simulink model "Controller"  (R2015a)
settings: Solver=ode3  SolverMode=SingleTasking  StartTime=0.0  StopTime=100  FixedStep=T_sim  RelTol=1e-3
PreLoadFcn:
  | LoadLibraries
values from neighbouring files (symbols this model uses):
  a = 10.26    [SetupComplete.m]
  A_x = 0.015    [SetupComplete.m]
  A_y = A_x    (= 0.015)    [SetupComplete.m]
  A_z = 0.16    [SetupComplete.m]
  C_d0 = 0.001193    [SetupComplete.m]
  C_x = 1.2    [SetupComplete.m]
  C_y = C_x    (= 1.2)    [SetupComplete.m]
  C_z = 2.2    [SetupComplete.m]
  CG_0 = [0,0,0.02]'    [SetupComplete.m]
  eta_23 = deg2rad(-1.42)    [Run3Copter.m]
  g = 9.81    [SetupComplete.m]
  h = 0.08    [SetupComplete.m]
  h_M = 0.064    [SetupComplete.m]
  I_BAC_0 = [ Ix,0,Ixz;0,Iy,0;Ixz,0,Iz]    [SetupComplete.m]
  Initial_Omegas = [1;1;1]*Omega_hover    [Run3Copter.m]
  l = 0.3450    (= 0.345)    [NDI_components.m]    (also in SetupComplete.m; robust_controller.m)
  l_arm = 0.264    [SetupComplete.m]
  m = 3.51    [SetupComplete.m]
  m_0 = 2.61    [SetupComplete.m]
  m_M = 0.300    (= 0.3)    [SetupComplete.m]
  R = 0.1778    [SetupComplete.m]    (also in robust_controller.m = eye(4))
  rho = 1.15    [SetupComplete.m]
  sigma = b*c/(pi*R)    (= 0.107416159567)    [SetupComplete.m]
  theta_0 = 0.38397    [SetupComplete.m]
  theta_1 = -0.2967    [SetupComplete.m]
  v_i0 = sqrt( 1/3*m*g/(2*rho*pi*R^2)  )    [SetupComplete.m]
undefined symbols (not defined in the file or in its folder): DOWN_0, EAST_0, Motor, NORTH_0, P_0, Prop, Q_0, R_0, Throttle_Hover, U_0, V_0, v_i_adim, Vx_adim, Vz_adim, W_0
undefined symbols (not defined in the file): Initial_Torques, J_FA, J_T, Rotation_sign, Tau_motors
libraries: XXCopter x39, simulink x35, vrlib x15, simulink_extras x7, aerolib6dofsys x2, qcatlib x2, dspinverses x2
(part 3 of 10)

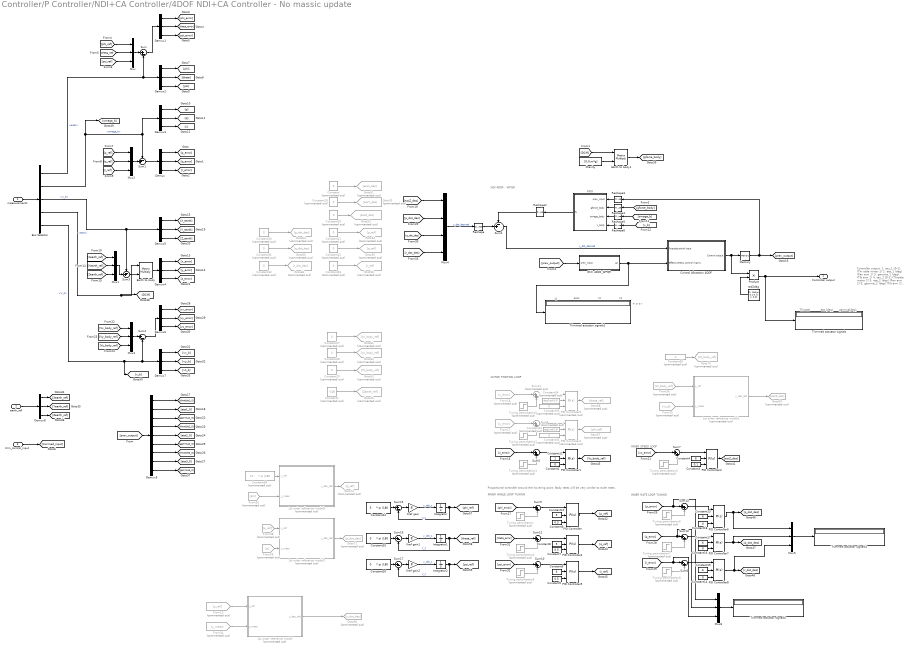
== system Controller/P Controller/NDI+CA Controller/4DOF NDI+CA Controller - No massic update ==
  note: NDI 4DOF - WPQR
  note: INNER SPEED LOOP
  note: INNER ANGLE LOOP TUNING
  note: INNER RATE LOOP TUNING
  note: Proportional controller around the hovering point. Body rates will be very similar to euler rates.
  note: Controller output:
      | 1. tau_1 [0-1] (Thr ottle motor 1)
      | 2. eta_1 (deg)  (Pan arm 1)
      | 3. gamma_1 (deg)  (Tilt arm 1)
      |
      | 4. tau_2 [0-1] (Throttle motor 2)
      | 5. eta_2 (deg)  (Pan arm 2)
      | 6. gamma_2 (deg)  (Tilt arm 2)
      |
      | 7. tau_3 [0-1] (Throttle motor 3)
      | 8. eta_3 (deg)  (Pan arm  3)
      | 9. gamma_3 (deg)  (Tilt arm 3)
  note: Throttle
  note: eta [deg]
  note: gamma[deg]
  note: OUTER POSITION LOOP
  note: eta1
  note: t3
  note: t2
  note: t1
  note: w
      | p
      | q
      | r
  measurements : Inport
  earth_ref : Inport  Port=2
  trim_control_input : Inport  Port=3
  1st order reference model : Subsystem  Commented=on  mask(1st order model reference block){Kref=1, Kb=20, fi=0.25, fc=0.5, Kf=1}
      mask prompts: Kref "1st order reference gain"; Kb "Bandwidth gain"; fi "Integral gain"; fc "Command FF gain"; Kf "Command_dot FF gain"
      mask help:
      | Generates a desired first order derivative of a commanded output taking
      | into account the current measured output.
      | Kref is the gain that determines the first order system between y_ref and
      | y_commanded signals. Ycom/Yref = Kref/(1 + Kref)
      | fi and fc can be defaulted to 0.25 and 0.5 for a critically damped 2nd
      | order response between y_meas and the error signal (y_com - y_meas) considering
      | a perfect dynamic inversion.
      mask Help:
      | Juan Herrero Macias <jn.herrerom@gmail.com>
      | This architecture can be found and explained in Fault-tolerant Flight
      | Control and Guidance Systems, Ducard, Guillaume.
      mask TypeOptions Kref: Kref gain/Gain
      mask TypeOptions Kb: Bandwidth gain/Gain
      mask TypeOptions fi: Integral gain/Gain
      mask TypeOptions fc: Command FF gain/Gain
      mask TypeOptions Kf: Command_dot FF gain/Gain
  1st order reference model1 : Subsystem  Commented=on  mask(1st order model reference block){Kref=2, Kb=2, fi=0.25, fc=0.5, Kf=1}
      mask prompts: Kref "1st order reference gain"; Kb "Bandwidth gain"; fi "Integral gain"; fc "Command FF gain"; Kf "Command_dot FF gain"
      mask help:
      | Generates a desired first order derivative of a commanded output taking
      | into account the current measured output.
      | Kref is the gain that determines the first order system between y_ref and
      | y_commanded signals. Ycom/Yref = Kref/(1 + Kref)
      | fi and fc can be defaulted to 0.25 and 0.5 for a critically damped 2nd
      | order response between y_meas and the error signal (y_com - y_meas) considering
      | a perfect dynamic inversion.
      mask Help:
      | Juan Herrero Macias <jn.herrerom@gmail.com>
      | This architecture can be found and explained in Fault-tolerant Flight
      | Control and Guidance Systems, Ducard, Guillaume.
      mask TypeOptions Kref: Kref gain/Gain
      mask TypeOptions Kb: Bandwidth gain/Gain
      mask TypeOptions fi: Integral gain/Gain
      mask TypeOptions fc: Command FF gain/Gain
      mask TypeOptions Kf: Command_dot FF gain/Gain
  1st order reference model2 : Subsystem  Commented=on  mask(1st order model reference block){Kref=2, Kb=2, fi=0.25, fc=0.5, Kf=1}
      mask prompts: Kref "1st order reference gain"; Kb "Bandwidth gain"; fi "Integral gain"; fc "Command FF gain"; Kf "Command_dot FF gain"
      mask help:
      | Generates a desired first order derivative of a commanded output taking
      | into account the current measured output.
      | Kref is the gain that determines the first order system between y_ref and
      | y_commanded signals. Ycom/Yref = Kref/(1 + Kref)
      | fi and fc can be defaulted to 0.25 and 0.5 for a critically damped 2nd
      | order response between y_meas and the error signal (y_com - y_meas) considering
      | a perfect dynamic inversion.
      mask Help:
      | Juan Herrero Macias <jn.herrerom@gmail.com>
      | This architecture can be found and explained in Fault-tolerant Flight
      | Control and Guidance Systems, Ducard, Guillaume.
      mask TypeOptions Kref: Kref gain/Gain
      mask TypeOptions Kb: Bandwidth gain/Gain
      mask TypeOptions fi: Integral gain/Gain
      mask TypeOptions fc: Command FF gain/Gain
      mask TypeOptions Kf: Command_dot FF gain/Gain
  1st order reference model3 : Subsystem  Commented=on  mask(1st order model reference block){Kref=2, Kb=2, fi=0.25, fc=0, Kf=0}
      mask prompts: Kref "1st order reference gain"; Kb "Bandwidth gain"; fi "Integral gain"; fc "Command FF gain"; Kf "Command_dot FF gain"
      mask help:
      | Generates a desired first order derivative of a commanded output taking
      | into account the current measured output.
      | Kref is the gain that determines the first order system between y_ref and
      | y_commanded signals. Ycom/Yref = Kref/(1 + Kref)
      | fi and fc can be defaulted to 0.25 and 0.5 for a critically damped 2nd
      | order response between y_meas and the error signal (y_com - y_meas) considering
      | a perfect dynamic inversion.
      mask Help:
      | Juan Herrero Macias <jn.herrerom@gmail.com>
      | This architecture can be found and explained in Fault-tolerant Flight
      | Control and Guidance Systems, Ducard, Guillaume.
      mask TypeOptions Kref: Kref gain/Gain
      mask TypeOptions Kb: Bandwidth gain/Gain
      mask TypeOptions fi: Integral gain/Gain
      mask TypeOptions fc: Command FF gain/Gain
      mask TypeOptions Kf: Command_dot FF gain/Gain
  Bus Selector : BusSelector  OutputSignals=euler,omega_b,X_e,DCM,V_b
  Constant{,19..23,27..33,35} (14 alike) : Constant  Commented=on  Value=0
  Constant1 : Constant  Commented=on  Value=-100
  Constant10 : Constant  Value=5
  Constant11 : Constant
  Constant12 : Constant  Commented=on  Value=deg2rad(0.5)
  Constant{4,13,15,17} (4 alike) : Constant  Value=6
  Constant{2,14,16,18} (4 alike) : Constant  Value=0
  Constant24 : Constant  Value="5     * pi /180"
  Constant25 : Constant  Value="0     * pi /180"
  Constant26 : Constant  Value="0     * pi /180"
  Constant3 : Constant  Value=0.1
  Constant34 : Constant  Commented=on  Value=-deg2rad(0.5)
  Constant36 : Constant  Commented=on  Value=-1
  Constant38 : Constant  Commented=on  Value="10     * pi /180"
  Constant5 : Constant  Value=0.5
  Constant6 : Constant  Value=5
  Constant7 : Constant  Value=0.5
  Constant8 : Constant  Value=5
  Constant9 : Constant  Value=0.5
  Control Allocation 4DOF : Subsystem  Variant=on  OverrideUsingVariant=(default)
  Demux{,1..8} (9 alike) : Demux  Outputs=3
  Demux9 : Demux  Outputs=9
  Earth to body : Product  Multiplication=Matrix(*)
  Earth to body1 : Product  Multiplication=Matrix(*)
  F(X) : MATLAB Function  TreatAsAtomicUnit=on
  From13 : From  Commented=on  GotoTag=y_ref
  From17 : From  Commented=on  GotoTag=y_error
  From18 : From  Commented=on  GotoTag=x_error
  From25 : From  Commented=on  GotoTag=vz_b
  From34 : From  Commented=on  GotoTag=y_meas
  From35 : From  Commented=on  GotoTag=phi
  From36 : From  Commented=on  GotoTag=Vz_body_ref
  From38 : From  Commented=on  GotoTag=p_ref
  From39 : From  Commented=on  GotoTag=p
  G(X) 4DOF_WPQR : MATLAB Function  TreatAsAtomicUnit=on
  Goto40 : Goto  Commented=on  GotoTag=Zearth_ref
  Goto51 : Goto  Commented=on  GotoTag=accX_des
  Goto52 : Goto  Commented=on  GotoTag=accY_des
  Goto53 : Goto  Commented=on  GotoTag=accZ_des
  Goto54 : Goto  Commented=on  GotoTag=p_ref
  Goto55 : Goto  Commented=on  GotoTag=q_ref
  Goto56 : Goto  Commented=on  GotoTag=r_ref
  Goto60 : Goto  Commented=on  GotoTag=y_dot_des
  Goto61 : Goto  Commented=on  GotoTag=Vx_body_ref
  Goto62 : Goto  Commented=on  GotoTag=Vy_body_ref
  Goto63 : Goto  Commented=on  GotoTag=Vz_body_ref
  Goto64 : Goto  Commented=on  GotoTag=p_dot_des
  Goto65 : Goto  Commented=on  GotoTag=q_dot_des
  Goto66 : Goto  Commented=on  GotoTag=r_dot_des
  Goto67 : Goto  Commented=on  GotoTag=phi_ref
  Goto68 : Goto  Commented=on  GotoTag=theta_ref
  Goto69 : Goto  Commented=on  GotoTag=accZ_des
  Goto70 : Goto  Commented=on  GotoTag=Vz_body_ref
  Goto71 : Goto  Commented=on  GotoTag=p_dot_des
  Goto72 : Goto  Commented=on  GotoTag=p_ref
  Gravity : Constant  Value=[0;0;m*g]
  Integrator : Integrator
  Integrator1 : Integrator
  Integrator2 : Integrator
  Kref gain : Gain  Gain=8
  Kref gain1 : Gain  Gain=8
  Kref gain2 : Gain  Gain=8
  Memory : Memory  X0=[0,0,0,0,0,0,0,0,0]  LinearizeAsDelay=on
  Mux{,1..3,5,8} (6 alike) : Mux  Inputs=3
  Mux4 : Mux
  PID Controller{,1..2,4..8} (8 alike) : simulink/Continuous/PID Controller  Controller=PI  TimeDomain=Continuous-time  SampleTime=-1  IntegratorMethod=Forward Euler  FilterMethod=Forward Euler  Form=Parallel  UseFilter=on  ControllerParametersSource=external  P=1  I=1  D=0  N=100  InitialConditionSource=internal  InitialConditionForIntegrator=0  InitialConditionForFilter=0  ExternalReset=none  LimitOutput=off  UpperSaturationLimit=inf  LowerSaturationLimit=-inf  LinearizeAsGain=on  AntiWindupMode=none  Kb=1  TrackingMode=off  Kt=1  PParamMin=[]  PParamMax=[]  IParamMin=[]  IParamMax=[]  DParamMin=[]  DParamMax=[]  NParamMin=[]  NParamMax=[]  KbParamMin=[]  KbParamMax=[]  KtParamMin=[]  KtParamMax=[]  POutMin=[]  POutMax=[]  IOutMin=[]  IOutMax=[]  DOutMin=[]  DOutMax=[]  NOutMin=[]  NOutMax=[]  KbOutMin=[]  KbOutMax=[]  KtOutMin=[]  KtOutMax=[]  IntegratorOutMin=[]  IntegratorOutMax=[]  FilterOutMin=[]  FilterOutMax=[]  SumOutMin=[]  SumOutMax=[]  SumI1OutMin=[]  SumI1OutMax=[]  SumI2OutMin=[]  SumI2OutMax=[]  SumI3OutMin=[]  SumI3OutMax=[]  SumDOutMin=[]  SumDOutMax=[]  SaturationOutMin=[]  SaturationOutMax=[]  IntegratorContinuousStateAttributes=''  IntegratorStateMustResolveToSignalObject=off  IntegratorRTWStateStorageClass=Auto  FilterContinuousStateAttributes=''  FilterStateMustResolveToSignalObject=off  FilterRTWStateStorageClass=Auto  DifferentiatorICPrevScaledInput=0  DifferentiatorOutMin=[]  DifferentiatorOutMax=[]
  PID Controller3 : simulink/Continuous/PID Controller  Commented=on  Controller=PI  TimeDomain=Continuous-time  SampleTime=-1  IntegratorMethod=Forward Euler  FilterMethod=Forward Euler  Form=Parallel  UseFilter=on  ControllerParametersSource=external  P=1  I=1  D=0  N=100  InitialConditionSource=internal  InitialConditionForIntegrator=0  InitialConditionForFilter=0  ExternalReset=none  LimitOutput=off  UpperSaturationLimit=inf  LowerSaturationLimit=-inf  LinearizeAsGain=on  AntiWindupMode=none  Kb=1  TrackingMode=off  Kt=1  PParamMin=[]  PParamMax=[]  IParamMin=[]  IParamMax=[]  DParamMin=[]  DParamMax=[]  NParamMin=[]  NParamMax=[]  KbParamMin=[]  KbParamMax=[]  KtParamMin=[]  KtParamMax=[]  POutMin=[]  POutMax=[]  IOutMin=[]  IOutMax=[]  DOutMin=[]  DOutMax=[]  NOutMin=[]  NOutMax=[]  KbOutMin=[]  KbOutMax=[]  KtOutMin=[]  KtOutMax=[]  IntegratorOutMin=[]  IntegratorOutMax=[]  FilterOutMin=[]  FilterOutMax=[]  SumOutMin=[]  SumOutMax=[]  SumI1OutMin=[]  SumI1OutMax=[]  SumI2OutMin=[]  SumI2OutMax=[]  SumI3OutMin=[]  SumI3OutMax=[]  SumDOutMin=[]  SumDOutMax=[]  SaturationOutMin=[]  SaturationOutMax=[]  IntegratorContinuousStateAttributes=''  IntegratorStateMustResolveToSignalObject=off  IntegratorRTWStateStorageClass=Auto  FilterContinuousStateAttributes=''  FilterStateMustResolveToSignalObject=off  FilterRTWStateStorageClass=Auto  DifferentiatorICPrevScaledInput=0  DifferentiatorOutMin=[]  DifferentiatorOutMax=[]
  PID Controller9 : simulink/Continuous/PID Controller  Commented=on  Controller=PI  TimeDomain=Continuous-time  SampleTime=-1  IntegratorMethod=Forward Euler  FilterMethod=Forward Euler  Form=Parallel  UseFilter=on  ControllerParametersSource=external  P=1  I=1  D=0  N=100  InitialConditionSource=internal  InitialConditionForIntegrator=0  InitialConditionForFilter=0  ExternalReset=none  LimitOutput=off  UpperSaturationLimit=inf  LowerSaturationLimit=-inf  LinearizeAsGain=on  AntiWindupMode=none  Kb=1  TrackingMode=off  Kt=1  PParamMin=[]  PParamMax=[]  IParamMin=[]  IParamMax=[]  DParamMin=[]  DParamMax=[]  NParamMin=[]  NParamMax=[]  KbParamMin=[]  KbParamMax=[]  KtParamMin=[]  KtParamMax=[]  POutMin=[]  POutMax=[]  IOutMin=[]  IOutMax=[]  DOutMin=[]  DOutMax=[]  NOutMin=[]  NOutMax=[]  KbOutMin=[]  KbOutMax=[]  KtOutMin=[]  KtOutMax=[]  IntegratorOutMin=[]  IntegratorOutMax=[]  FilterOutMin=[]  FilterOutMax=[]  SumOutMin=[]  SumOutMax=[]  SumI1OutMin=[]  SumI1OutMax=[]  SumI2OutMin=[]  SumI2OutMax=[]  SumI3OutMin=[]  SumI3OutMax=[]  SumDOutMin=[]  SumDOutMax=[]  SaturationOutMin=[]  SaturationOutMax=[]  IntegratorContinuousStateAttributes=''  IntegratorStateMustResolveToSignalObject=off  IntegratorRTWStateStorageClass=Auto  FilterContinuousStateAttributes=''  FilterStateMustResolveToSignalObject=off  FilterRTWStateStorageClass=Auto  DifferentiatorICPrevScaledInput=0  DifferentiatorOutMin=[]  DifferentiatorOutMax=[]
  Product : Product
  Reshape : Reshape  OutputDimensionality=Column vector (2-D)
  Reshape2 : Reshape  OutputDimensionality=Column vector (2-D)  OutputDimensions=[6,1]
  Reshape{3..6} (4 alike) : Reshape  OutputDimensions=[6,1]
  Sum{,4,15..17} (5 alike) : Sum  Inputs=|+-
  Sum1 : Sum  Inputs=-+|
  Sum{5,7..10,12..14} (8 alike) : Sum  Inputs=|++
  Sum11 : Sum  Commented=on  Inputs=|++
  Sum2 : Sum  Inputs=-+|
  Sum3 : Sum  Inputs=-+|
  Sum6 : Sum  Commented=on  Inputs=|++
  Trimmed actuator signals{,1,3,5} (4 alike) : Display
  Tuning perturbation{,5..6,8} (4 alike) : Step  Commented=on  Time=20  After=3*pi/180  SampleTime=0
  Tuning perturbation{1..3,9} (4 alike) : Step  Commented=on  Time=20  SampleTime=0
  Tuning perturbation4 : Step  Commented=on  Time=20  After=-3*pi/180  SampleTime=0
  Tuning perturbation7 : Step  Commented=on  Time=20  After=-3*pi/180  SampleTime=0
  rad2deg : Constant  Value=[1, 180/pi, 0,1,0, 0, 1, 0,0]
  Controller output : Outport
  wires:
  Demux9/9 -> [gamma3_0]
  Demux9/8 -> [eta3_0]
  Demux9/7 -> [throttle3_0]
  Demux9/6 -> [gamma2_0]
  Demux9/5 -> [eta2_0]
  Demux9/4 -> [throttle2_0]
  Demux9/3 -> [gamma1_0]
  Demux9/2 -> [eta1_0]
  Demux9/1 -> [throttle1_0]
  [prev_output] -> Demux9/1
  earth_ref/1 -> Demux8/1
  Demux8/1 -> [Xearth_ref]
  Demux8/2 -> [Yearth_ref]
  Demux8/3 -> [Zearth_ref]
  Earth to body/1 -> Demux4/1
  Bus Selector/4 -> Earth to body/1, [DCM]  "<DCM>"
  [Vz_body_ref] -> Mux3/3
  [Vx_body_ref] -> Mux3/1
  [Vy_body_ref] -> Mux3/2
  Demux6/3 -> [vz_error]
  Demux6/2 -> [vy_error]
  Demux6/1 -> [vx_error]
  Sum4/1 -> Demux6/1
  Bus Selector/5 -> [v_b], Sum4/2, Demux7/1  "<V_b>"
  Demux7/3 -> [vz_b]
  Demux7/2 -> [vy_b]
  Demux7/1 -> [vx_b]
  Mux3/1 -> Sum4/1
  [Zearth_ref] -> Mux1/3
  [Xearth_ref] -> Mux1/1
  [Yearth_ref] -> Mux1/2
  Mux1/1 -> Sum3/2
  Demux4/1 -> [x_error]
  Demux4/2 -> [y_error]
  Demux4/3 -> [z_error]
  Demux5/1 -> [X_earth]
  Demux5/2 -> [Y_earth]
  Demux5/3 -> [Z_earth]
  Bus Selector/3 -> Sum3/1, Demux5/1  "<X_e>"
  [r_ref] -> Mux2/3
  [p_ref] -> Mux2/1
  [q_ref] -> Mux2/2
  Mux2/1 -> Sum1/2
  [psi_ref] -> Mux/3
  [phi_ref] -> Mux/1
  [theta_ref] -> Mux/2
  trim_control_input/1 -> [trimmed_input]
  Demux1/3 -> [psi_error]
  Demux1/2 -> [theta_error]
  Demux1/1 -> [phi_error]
  Demux/1 -> [p_error]
  Demux/2 -> [q_error]
  Demux/3 -> [r_error]
  Sum/1 -> Demux1/1
  Sum1/1 -> Demux/1
  Bus Selector/2 -> [omega_b], Sum1/1, Demux3/1  "<omega_b>"
  Bus Selector/1 -> Sum/2, Demux2/1  "<euler>"
  measurements/1 -> Bus Selector/1
  Demux2/3 -> [psi]
  Demux2/2 -> [theta]
  Demux2/1 -> [phi]
  Demux3/1 -> [p]
  Demux3/2 -> [q]
  Demux3/3 -> [r]
  Mux/1 -> Sum/1
  F(X)/1(fx) -> Reshape2/1
  Gravity/1 -> Earth to body1/2
  Earth to body1/1 -> [gforce_body]
  [gforce_body] -> Reshape4/1
  Constant4/1 -> PID Controller2/2
  Constant3/1 -> PID Controller2/3
  Sum7/1 -> PID Controller2/1
  [vz_error] -> Sum7/1
  Tuning perturbation3/1 -> Sum7/2
  PID Controller/1 -> [p_ref]
  PID Controller4/1 -> [q_ref]
  PID Controller5/1 -> [r_ref]
  Constant6/1 -> PID Controller5/2
  Constant5/1 -> PID Controller5/3
  Constant8/1 -> PID Controller4/2
  Constant10/1 -> PID Controller/2
  Constant9/1 -> PID Controller/3
  Constant7/1 -> PID Controller4/3
  Sum9/1 -> PID Controller/1
  Sum10/1 -> PID Controller5/1
  Sum12/1 -> PID Controller4/1
  Tuning perturbation5/1 -> Sum10/2
  Tuning perturbation/1 -> Sum9/2
  Tuning perturbation4/1 -> Sum12/2
  PID Controller6/1 -> Mux5/1, [p_dot_des]
  PID Controller7/1 -> Mux5/2, [q_dot_des]
  PID Controller8/1 -> Mux5/3, [r_dot_des]
  Constant15/1 -> PID Controller8/2
  Constant14/1 -> PID Controller8/3
  Constant17/1 -> PID Controller7/2
  Constant16/1 -> PID Controller7/3
  Sum14/1 -> PID Controller6/1
  Sum8/1 -> PID Controller8/1
  Sum13/1 -> PID Controller7/1
  Tuning perturbation8/1 -> Sum8/2
  Tuning perturbation6/1 -> Sum14/2
  Tuning perturbation7/1 -> Sum13/2
  Mux4/1 -> Reshape/1  "y_dot_desired"
  Reshape/1 -> Sum2/2
  Reshape2/1 -> Sum2/1
  Reshape3/1 -> F(X)/1(prev_input)
  [omega_b] -> Reshape5/1
  Reshape4/1 -> F(X)/2(gforce_body)
  Reshape5/1 -> F(X)/3(omega_body)
  Reshape6/1 -> F(X)/4(v_body)
  [v_b] -> Reshape6/1
  Constant/1 -> Goto51/1
  Constant19/1 -> Goto52/1
  Constant20/1 -> Goto53/1
  Constant21/1 -> Goto54/1
  Constant22/1 -> Goto55/1
  Constant23/1 -> Goto56/1
  Constant18/1 -> PID Controller6/3
  Product/1 -> Trimmed actuator signals/1, Controller output/1
  rad2deg/1 -> Product/2
  From13/1 -> 1st order reference model/1(y_ref)
  From34/1 -> 1st order reference model/2(y_meas)
  1st order reference model/1(y_des_dot) -> Goto60/1
  Mux5/1 -> Trimmed actuator signals3/1
  PID Controller2/1 -> [accZ_des]
  Constant27/1 -> Goto61/1
  Constant28/1 -> Goto62/1
  Constant29/1 -> Goto63/1
  [phi_error] -> Sum9/1
  [theta_error] -> Sum12/1
  [psi_error] -> Sum10/1
  [p_error] -> Mux8/1, Sum14/1
  [q_error] -> Mux8/2, Sum13/1
  [r_error] -> Mux8/3, Sum8/1
  Mux8/1 -> Trimmed actuator signals5/1
  [DCM] -> Earth to body1/1
  Memory/1 -> Reshape3/1, [prev_output]
  Constant30/1 -> Goto64/1
  Constant31/1 -> Goto65/1
  Constant32/1 -> Goto66/1
  Sum3/1 -> Earth to body/2
  Constant13/1 -> PID Controller6/2
  Sum2/1 -> Control Allocation 4DOF/1(Pseudocontrol input)  "y_dot_desired"
  Control Allocation 4DOF/1(Control output) -> Product/1, Memory/1
  [prev_output] -> G(X) 4DOF_WPQR/1(prev_input)
  [accZ_des] -> Mux4/1
  [p_dot_des] -> Mux4/2
  [q_dot_des] -> Mux4/3
  [r_dot_des] -> Mux4/4
  Constant1/1 -> Goto40/1
  Constant11/1 -> PID Controller1/2
  Constant2/1 -> PID Controller1/3
  Sum5/1 -> PID Controller1/1
  [z_error] -> Sum5/1
  Tuning perturbation1/1 -> Sum5/2
  PID Controller1/1 -> [Vz_body_ref]
  Constant12/1 -> PID Controller3/2
  Constant33/1 -> PID Controller3/3
  Sum6/1 -> PID Controller3/1
  From17/1 -> Sum6/1
  Tuning perturbation2/1 -> Sum6/2
  PID Controller3/1 -> Goto67/1
  Constant34/1 -> PID Controller9/2
  Constant35/1 -> PID Controller9/3
  Sum11/1 -> PID Controller9/1
  From18/1 -> Sum11/1
  Tuning perturbation9/1 -> Sum11/2
  PID Controller9/1 -> Goto68/1
  G(X) 4DOF_WPQR/1(gx) -> Trimmed actuator signals1/1, Control Allocation 4DOF/2(Effectiveness control matrix)
  From36/1 -> 1st order reference model1/1(y_ref)
  From25/1 -> 1st order reference model1/2(y_meas)
  1st order reference model1/1(y_des_dot) -> Goto69/1
  Constant36/1 -> Goto70/1
  From39/1 -> 1st order reference model2/2(y_meas)
  1st order reference model2/1(y_des_dot) -> Goto71/1
  From38/1 -> 1st order reference model2/1(y_ref)
  From35/1 -> 1st order reference model3/2(y_meas)
  1st order reference model3/1(y_des_dot) -> Goto72/1
  Constant38/1 -> 1st order reference model3/1(y_ref)
  Constant24/1 -> Sum15/1
  Integrator/1 -> Sum15/2, [phi_ref]  "y_c"
  Kref gain/1 -> Integrator/1  "y_dot_c"
  Sum15/1 -> Kref gain/1
  Constant25/1 -> Sum16/1
  Integrator1/1 -> [theta_ref], Sum16/2  "y_c"
  Kref gain1/1 -> Integrator1/1  "y_dot_c"
  Sum16/1 -> Kref gain1/1
  Constant26/1 -> Sum17/1
  Integrator2/1 -> Sum17/2, [psi_ref]  "y_c"
  Kref gain2/1 -> Integrator2/1  "y_dot_c"
  Sum17/1 -> Kref gain2/1

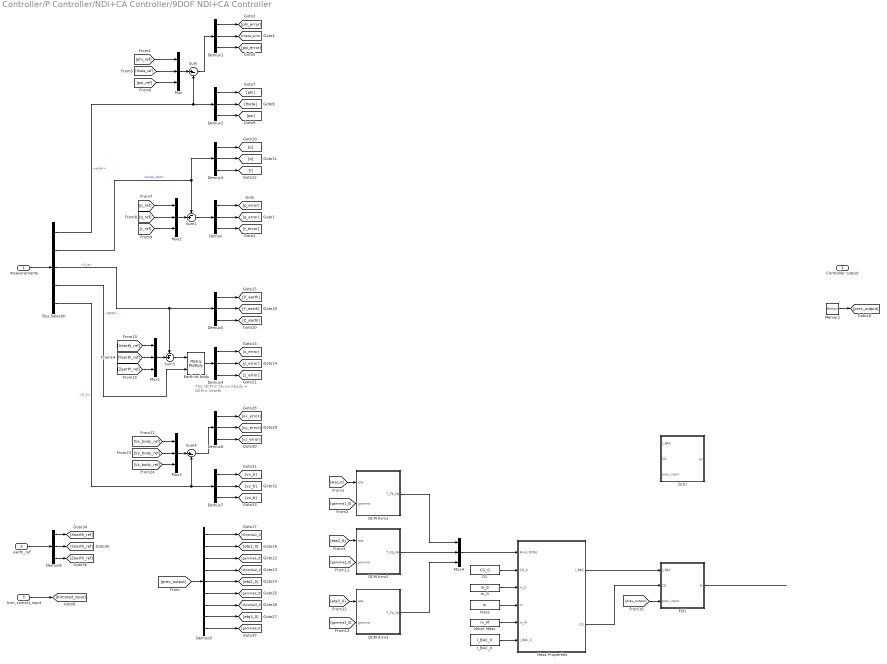
== system Controller/P Controller/NDI+CA Controller/9DOF NDI+CA Controller ==
  note: This DCM is Tb->e
      | Xbody = DCM x Xearth
  measurements : Inport
  earth_ref : Inport  Port=2
  trim_control_input : Inport  Port=3
  Bus Selector : BusSelector  OutputSignals=euler,euler_dot,X_e,DCM,V_b
  CG : Constant  Value=CG_0
  DCM Arm1 : MATLAB Function  TreatAsAtomicUnit=on
  DCM Arm2 : MATLAB Function  TreatAsAtomicUnit=on
  DCM Arm3 : MATLAB Function  TreatAsAtomicUnit=on
  Demux{,1..8} (9 alike) : Demux  Outputs=3
  Demux9 : Demux  Outputs=9
  Earth to body : Product  Multiplication=Matrix(*)
  F(X) : MATLAB Function  TreatAsAtomicUnit=on
  G(X) : MATLAB Function  TreatAsAtomicUnit=on
  I_BAC_0 : Constant  Value=I_BAC_0
  Mass Properties : Subsystem  TreatAsAtomicUnit=on
  Memory : Memory  LinearizeAsDelay=on
  Motor Mass : Constant  Value=m_M
  Mux{,1..4} (5 alike) : Mux  Inputs=3
  Sum : Sum  Inputs=|+-
  Sum1 : Sum  Inputs=-+|
  Sum3 : Sum  Inputs=-+|
  Sum4 : Sum  Inputs=|+-
  m_0 : Constant  Value=m_0
  mass : Constant  Value=m
  Controller output : Outport
  wires:
  Mux/1 -> Sum/1
  Demux3/3 -> [r]
  Demux3/2 -> [q]
  Demux3/1 -> [p]
  Demux2/1 -> [phi]
  Demux2/2 -> [theta]
  Demux2/3 -> [psi]
  measurements/1 -> Bus Selector/1
  Bus Selector/1 -> Demux2/1, Sum/2  "<euler>"
  Bus Selector/2 -> Demux3/1, Sum1/1  "<euler_dot>"
  Sum1/1 -> Demux/1
  Sum/1 -> Demux1/1
  Demux/3 -> [r_error]
  Demux/2 -> [q_error]
  Demux/1 -> [p_error]
  Demux1/1 -> [phi_error]
  Demux1/2 -> [theta_error]
  Demux1/3 -> [psi_error]
  trim_control_input/1 -> [trimmed_input]
  [theta_ref] -> Mux/2
  [phi_ref] -> Mux/1
  [psi_ref] -> Mux/3
  Mux2/1 -> Sum1/2
  [q_ref] -> Mux2/2
  [p_ref] -> Mux2/1
  [r_ref] -> Mux2/3
  Bus Selector/3 -> Demux5/1, Sum3/1  "<X_e>"
  Demux5/3 -> [Z_earth]
  Demux5/2 -> [Y_earth]
  Demux5/1 -> [X_earth]
  Demux4/3 -> [z_error]
  Demux4/2 -> [y_error]
  Demux4/1 -> [x_error]
  Mux1/1 -> Sum3/2
  [Yearth_ref] -> Mux1/2
  [Xearth_ref] -> Mux1/1
  [Zearth_ref] -> Mux1/3
  Mux3/1 -> Sum4/1
  Demux7/1 -> [vx_b]
  Demux7/2 -> [vy_b]
  Demux7/3 -> [vz_b]
  Bus Selector/5 -> Demux7/1, Sum4/2  "<V_b>"
  Sum4/1 -> Demux6/1
  Demux6/1 -> [vx_error]
  Demux6/2 -> [vy_error]
  Demux6/3 -> [vz_error]
  [Vy_body_ref] -> Mux3/2
  [Vx_body_ref] -> Mux3/1
  [Vz_body_ref] -> Mux3/3
  Bus Selector/4 -> Earth to body/2  "<DCM>"
  Earth to body/1 -> Demux4/1
  Sum3/1 -> Earth to body/1
  Demux8/3 -> [Zearth_ref]
  Demux8/2 -> [Yearth_ref]
  Demux8/1 -> [Xearth_ref]
  earth_ref/1 -> Demux8/1
  ? -> Controller output/1, Memory/1
  Memory/1 -> [prev_output]
  [prev_output] -> Demux9/1
  Demux9/1 -> [throttle1_0]
  Demux9/2 -> [eta1_0]
  Demux9/3 -> [gamma1_0]
  Demux9/4 -> [throttle2_0]
  Demux9/5 -> [eta2_0]
  Demux9/6 -> [gamma2_0]
  Demux9/7 -> [throttle3_0]
  Demux9/8 -> [eta3_0]
  Demux9/9 -> [gamma3_0]
  [eta1_0] -> DCM Arm1/1(eta)
  [gamma1_0] -> DCM Arm1/2(gamma)
  [eta2_0] -> DCM Arm2/1(eta)
  [gamma2_0] -> DCM Arm2/2(gamma)
  [eta3_0] -> DCM Arm3/1(eta)
  [gamma3_0] -> DCM Arm3/2(gamma)
  CG/1 -> Mass Properties/2(CG_0)
  Motor Mass/1 -> Mass Properties/5(m_M)
  I_BAC_0/1 -> Mass Properties/6(I_BAC_0)
  m_0/1 -> Mass Properties/3(m_0)
  mass/1 -> Mass Properties/4(m)
  Mux4/1 -> Mass Properties/1(Arms DCMs)
  DCM Arm1/1(T_Fb_FA) -> Mux4/1
  DCM Arm2/1(T_Fb_FA) -> Mux4/2
  DCM Arm3/1(T_Fb_FA) -> Mux4/3
  Mass Properties/1(I_BAC) -> F(X)/1(I_BAC)
  Mass Properties/2(CG) -> F(X)/2(CG)
  [prev_output] -> F(X)/3(prev_input)
  F(X)/1(fx) -> ?

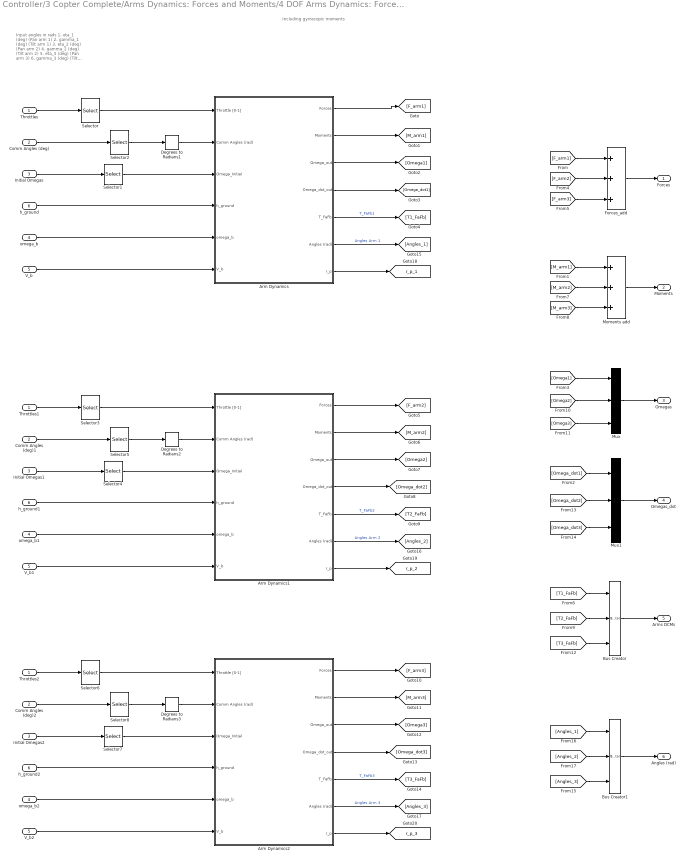
== system Controller/3 Copter Complete/Arms Dynamics: Forces and Moments/4 DOF Arms Dynamics: Forces and Moments1/4 DOF Arms Dynamics: Forces and Moments1 ==
  note: Including gyroscopic moments
  note: Input angles in rads
      |
      | 1. eta_1 (deg)  (Pan arm 1)
      | 2. gamma_1 (deg)  (Tilt arm 1)
      |
      | 3. eta_2 (deg)  (Pan arm 2)
      | 4. gamma_2 (deg)  (Tilt arm 2)
      |
      | 5. eta_3 (deg)  (Pan arm  3)
      | 6. gamma_3 (deg)  (Tilt arm 3)
  Throttles : Inport
  Comm Angles (deg) : Inport  Port=2
  Initial Omegas : Inport  Port=3
  omega_b : Inport  Port=4
  V_b : Inport  Port=5
  h_ground : Inport  Port=6
  Arm Dynamics : Subsystem  AncestorBlock=XXCopter/Arm Dynamics  TreatAsAtomicUnit=on  mask(Arm dynamics, kinematics, forces and moments){Rot_sign=Rotation_sign(1), tau=Tau_motors, arm_hub_pos=l*[1;0;0], arm_axis=[l_arm;0;0], arm_num=1, eta_dir=[1;0;0], gamma_dir=[0;1;0], J_T=J_T, J_FA=J_FA, h=h, Torq_ini=Initial_Torques(1), Omega_ini=Initial_Omegas(1), init_eta=0, init_gamma=0, omega_n=35, xi=1.45, c=0.01}
      mask prompts: Rot_sign "Rotation sign"; tau "Tau motors"; arm_hub_pos "Arm Hub position"; arm_axis "Arm Hub from servo"; arm_num "Arm number"; eta_dir "eta direcction"; gamma_dir "gamma direction"; J_T "Inertia Motor+prop"; J_FA "Inertia Forearm"; h "h propeller hub"; Torq_ini "Torque Initial Condition"; Omega_ini "Omega Initial Condition"; init_eta "Initial eta  (rad)"; init_gamma "Initial gamma  (rad)"; omega_n "Servo natural frequency"; xi "Servo damping"; c "Derivative param"
      mask help:
      | This block only accepts arms oriented in x-axis or y-axis: eta and gamma directions can only be [1,0,0] or [0,1,0]
      | Note rotations order is [eta (pan) ,gamma (tilt),0]
      |
      | If Arm number 1 (Forward one)
      | eta_dir=[1,0,0]
      | gamma_dir=[0,1,0]
      |
      | If Arm number 2 or 3 (rear ones)
      | eta_dir=[0,1,0]
      | gamma_dir=[1,0,0]
      mask TypeOptions Rot_sign: Aerodynamics Propeller/Rot_sign | Gyroscopic Moments/Rot_sign
      mask TypeOptions tau: ESC+Motor Dynamcis/tau
      mask TypeOptions arm_hub_pos: Arms Kinematics/Arm_hub_position
      mask TypeOptions arm_axis: Gyroscopic Moments/Arm_axis
      mask TypeOptions arm_num: Arms Kinematics/Arm_number
      mask TypeOptions eta_dir: Arms Kinematics/eta_dir | Gyroscopic Moments/eta_dir
      mask TypeOptions gamma_dir: Arms Kinematics/gamma_dir | Gyroscopic Moments/gamma_dir
      mask TypeOptions J_T: ESC+Motor Dynamcis/J_T | Gyroscopic Moments/J_T
      mask TypeOptions J_FA: Gyroscopic Moments/J_FA
      mask TypeOptions h: Arms Kinematics/h_prop
      mask TypeOptions Torq_ini: Initial_torque/X0
      mask TypeOptions Omega_ini: initial_omega/X0
      mask TypeOptions init_eta: Servos Dynamics/init_eta
      mask TypeOptions omega_n: Servos Dynamics/omega_n
      mask TypeOptions xi: Servos Dynamics/xi
      mask TypeOptions c: Servos Dynamics/derv_param
      mask Display:
      | % fprintf(' Arm number %i \n dynamics',arm_num)
      | 
      | 
      | disp(['{\bf \fontsize{16}',sprintf('Arm number\n\n'),num2str(arm_num),sprintf('\n\n Dynamics '),'}'], 'texmode','on');
  Arm Dynamics1 : Subsystem  AncestorBlock=XXCopter/Arm Dynamics  TreatAsAtomicUnit=on  mask(Arm dynamics, kinematics, forces and moments){Rot_sign=Rotation_sign(2), tau=Tau_motors, arm_hub_pos=l*[-1/2;sqrt(3)/2;0], arm_axis=[0;l_arm;0], arm_num=2, eta_dir=[0;1;0], gamma_dir=[1;0;0], J_T=J_T, J_FA=J_FA, h=h, Torq_ini=Initial_Torques(2), Omega_ini=Initial_Omegas(2), init_eta=0, init_gamma=0, omega_n=35, xi=1.45, c=0.01}
      mask prompts: Rot_sign "Rotation sign"; tau "Tau motors"; arm_hub_pos "Arm Hub position"; arm_axis "Arm Hub from servo"; arm_num "Arm number"; eta_dir "eta direcction"; gamma_dir "gamma direction"; J_T "Inertia Motor+prop"; J_FA "Inertia Forearm"; h "h propeller hub"; Torq_ini "Torque Initial Condition"; Omega_ini "Omega Initial Condition"; init_eta "Initial eta  (rad)"; init_gamma "Initial gamma  (rad)"; omega_n "Servo natural frequency"; xi "Servo damping"; c "Derivative param"
      mask help:
      | This block only accepts arms oriented in x-axis or y-axis: eta and gamma directions can only be [1,0,0] or [0,1,0]
      | Note rotations order is [eta (pan) ,gamma (tilt),0]
      |
      | If Arm number 1 (Forward one)
      | eta_dir=[1,0,0]
      | gamma_dir=[0,1,0]
      |
      | If Arm number 2 or 3 (rear ones)
      | eta_dir=[0,1,0]
      | gamma_dir=[1,0,0]
      mask TypeOptions Rot_sign: Aerodynamics Propeller/Rot_sign | Gyroscopic Moments/Rot_sign
      mask TypeOptions tau: ESC+Motor Dynamcis/tau
      mask TypeOptions arm_hub_pos: Arms Kinematics/Arm_hub_position
      mask TypeOptions arm_axis: Gyroscopic Moments/Arm_axis
      mask TypeOptions arm_num: Arms Kinematics/Arm_number
      mask TypeOptions eta_dir: Arms Kinematics/eta_dir | Gyroscopic Moments/eta_dir
      mask TypeOptions gamma_dir: Arms Kinematics/gamma_dir | Gyroscopic Moments/gamma_dir
      mask TypeOptions J_T: ESC+Motor Dynamcis/J_T | Gyroscopic Moments/J_T
      mask TypeOptions J_FA: Gyroscopic Moments/J_FA
      mask TypeOptions h: Arms Kinematics/h_prop
      mask TypeOptions Torq_ini: Initial_torque/X0
      mask TypeOptions Omega_ini: initial_omega/X0
      mask TypeOptions init_eta: Servos Dynamics/init_eta
      mask TypeOptions omega_n: Servos Dynamics/omega_n
      mask TypeOptions xi: Servos Dynamics/xi
      mask TypeOptions c: Servos Dynamics/derv_param
      mask Display:
      | % fprintf(' Arm number %i \n dynamics',arm_num)
      | 
      | 
      | disp(['{\bf \fontsize{16}',sprintf('Arm number\n\n'),num2str(arm_num),sprintf('\n\n Dynamics '),'}'], 'texmode','on');
  Arm Dynamics2 : Subsystem  AncestorBlock=XXCopter/Arm Dynamics  TreatAsAtomicUnit=on  mask(Arm dynamics, kinematics, forces and moments){Rot_sign=Rotation_sign(3), tau=Tau_motors, arm_hub_pos=l*[-1/2;-sqrt(3)/2;0], arm_axis=[0;-l_arm;0], arm_num=3, eta_dir=[0;1;0], gamma_dir=[1;0;0], J_T=J_T, J_FA=J_FA, h=h, Torq_ini=Initial_Torques(3), Omega_ini=Initial_Omegas(3), init_eta=0, init_gamma=0, omega_n=35, xi=1.45, c=0.01}
      mask prompts: Rot_sign "Rotation sign"; tau "Tau motors"; arm_hub_pos "Arm Hub position"; arm_axis "Arm Hub from servo"; arm_num "Arm number"; eta_dir "eta direcction"; gamma_dir "gamma direction"; J_T "Inertia Motor+prop"; J_FA "Inertia Forearm"; h "h propeller hub"; Torq_ini "Torque Initial Condition"; Omega_ini "Omega Initial Condition"; init_eta "Initial eta  (rad)"; init_gamma "Initial gamma  (rad)"; omega_n "Servo natural frequency"; xi "Servo damping"; c "Derivative param"
      mask help:
      | This block only accepts arms oriented in x-axis or y-axis: eta and gamma directions can only be [1,0,0] or [0,1,0]
      | Note rotations order is [eta (pan) ,gamma (tilt),0]
      |
      | If Arm number 1 (Forward one)
      | eta_dir=[1,0,0]
      | gamma_dir=[0,1,0]
      |
      | If Arm number 2 or 3 (rear ones)
      | eta_dir=[0,1,0]
      | gamma_dir=[1,0,0]
      mask TypeOptions Rot_sign: Aerodynamics Propeller/Rot_sign | Gyroscopic Moments/Rot_sign
      mask TypeOptions tau: ESC+Motor Dynamcis/tau
      mask TypeOptions arm_hub_pos: Arms Kinematics/Arm_hub_position
      mask TypeOptions arm_axis: Gyroscopic Moments/Arm_axis
      mask TypeOptions arm_num: Arms Kinematics/Arm_number
      mask TypeOptions eta_dir: Arms Kinematics/eta_dir | Gyroscopic Moments/eta_dir
      mask TypeOptions gamma_dir: Arms Kinematics/gamma_dir | Gyroscopic Moments/gamma_dir
      mask TypeOptions J_T: ESC+Motor Dynamcis/J_T | Gyroscopic Moments/J_T
      mask TypeOptions J_FA: Gyroscopic Moments/J_FA
      mask TypeOptions h: Arms Kinematics/h_prop
      mask TypeOptions Torq_ini: Initial_torque/X0
      mask TypeOptions Omega_ini: initial_omega/X0
      mask TypeOptions init_eta: Servos Dynamics/init_eta
      mask TypeOptions omega_n: Servos Dynamics/omega_n
      mask TypeOptions xi: Servos Dynamics/xi
      mask TypeOptions c: Servos Dynamics/derv_param
      mask Display:
      | % fprintf(' Arm number %i \n dynamics',arm_num)
      | 
      | 
      | disp(['{\bf \fontsize{16}',sprintf('Arm number\n\n'),num2str(arm_num),sprintf('\n\n Dynamics '),'}'], 'texmode','on');
  Bus Creator : BusCreator  Inputs=3
  Bus Creator1 : BusCreator  Inputs=3
  Comm Angles (deg)1 : InportShadow  Port=2
  Comm Angles (deg)2 : InportShadow  Port=2
  Degrees to Radians1 : simulink_extras/Transformations/Degrees to Radians
  Degrees to Radians2 : simulink_extras/Transformations/Degrees to Radians
  Degrees to Radians3 : simulink_extras/Transformations/Degrees to Radians
  Forces_add : Sum  Inputs=+++
  Initial Omegas1 : InportShadow  Port=3
  Initial Omegas2 : InportShadow  Port=3
  Moments add : Sum  Inputs=+++
  Mux : Mux  Inputs=3
  Mux1 : Mux  Inputs=3
  Selector : Selector  InputPortWidth=3  Indices=[1]
  Selector1 : Selector  InputPortWidth=3  Indices=[1]
  Selector2 : Selector  InputPortWidth=6  Indices=[1,2]
  Selector3 : Selector  InputPortWidth=3  Indices=2
  Selector4 : Selector  InputPortWidth=3  Indices=2
  Selector5 : Selector  InputPortWidth=6  Indices=[3,4]
  Selector6 : Selector  InputPortWidth=3  Indices=3
  Selector7 : Selector  InputPortWidth=3  Indices=3
  Selector8 : Selector  InputPortWidth=6  Indices=[5,6]
  Throttles1 : InportShadow
  Throttles2 : InportShadow
  V_b1 : InportShadow  Port=5
  V_b2 : InportShadow  Port=5
  h_ground1 : InportShadow  Port=6
  h_ground2 : InportShadow  Port=6
  omega_b1 : InportShadow  Port=4
  omega_b2 : InportShadow  Port=4
  Forces : Outport
  Moments : Outport  Port=2
  Omegas : Outport  Port=3
  Omegas_dot : Outport  Port=4
  Arms DCMs : Outport  Port=5
  Angles (rad) : Outport  Port=6
  tag scope: r_p_1=global, r_p_2=global, r_p_3=global
  wires:
  Selector1/1 -> Arm Dynamics/3(Omega_Initial)
  Throttles/1 -> Selector/1
  Initial Omegas/1 -> Selector1/1
  Selector/1 -> Arm Dynamics/1(Throttle [0-1])
  V_b/1 -> Arm Dynamics/6(V_b)
  Forces_add/1 -> Forces/1
  Moments add/1 -> Moments/1
  Mux/1 -> Omegas/1
  Mux1/1 -> Omegas_dot/1
  h_ground/1 -> Arm Dynamics/4(h_ground)
  Arm Dynamics/1(Forces) -> [F_arm1]
  Arm Dynamics/2(Moments) -> [M_arm1]
  Arm Dynamics/3(Omega_out) -> [Omega1]
  Arm Dynamics/4(Omega_dot_out) -> [Omega_dot1]
  [F_arm1] -> Forces_add/1
  [M_arm1] -> Moments add/1
  [Omega_dot1] -> Mux1/1
  [Omega1] -> Mux/1
  omega_b/1 -> Arm Dynamics/5(omega_b)
  [F_arm2] -> Forces_add/2
  [F_arm3] -> Forces_add/3
  [Omega2] -> Mux/2
  [Omega3] -> Mux/3
  [Omega_dot2] -> Mux1/2
  [Omega_dot3] -> Mux1/3
  [M_arm3] -> Moments add/3
  [M_arm2] -> Moments add/2
  Degrees to Radians1/1 -> Arm Dynamics/2(Comm Angles (rad))
  Comm Angles (deg)/1 -> Selector2/1
  Selector2/1 -> Degrees to Radians1/1
  Arm Dynamics/5(T_FaFb) -> [T1_FaFb]  "T_FaFb1"
  Bus Creator/1 -> Arms DCMs/1
  [T1_FaFb] -> Bus Creator/1
  Selector4/1 -> Arm Dynamics1/3(Omega_Initial)
  Throttles1/1 -> Selector3/1
  Initial Omegas1/1 -> Selector4/1
  Selector3/1 -> Arm Dynamics1/1(Throttle [0-1])
  V_b1/1 -> Arm Dynamics1/6(V_b)
  h_ground1/1 -> Arm Dynamics1/4(h_ground)
  Arm Dynamics1/1(Forces) -> [F_arm2]
  Arm Dynamics1/2(Moments) -> [M_arm2]
  Arm Dynamics1/3(Omega_out) -> [Omega2]
  Arm Dynamics1/4(Omega_dot_out) -> [Omega_dot2]
  omega_b1/1 -> Arm Dynamics1/5(omega_b)
  Degrees to Radians2/1 -> Arm Dynamics1/2(Comm Angles (rad))
  Comm Angles (deg)1/1 -> Selector5/1
  Selector5/1 -> Degrees to Radians2/1
  Arm Dynamics1/5(T_FaFb) -> [T2_FaFb]  "T_FaFb2"
  [T2_FaFb] -> Bus Creator/2
  Selector7/1 -> Arm Dynamics2/3(Omega_Initial)
  Throttles2/1 -> Selector6/1
  Initial Omegas2/1 -> Selector7/1
  Selector6/1 -> Arm Dynamics2/1(Throttle [0-1])
  V_b2/1 -> Arm Dynamics2/6(V_b)
  h_ground2/1 -> Arm Dynamics2/4(h_ground)
  Arm Dynamics2/1(Forces) -> [F_arm3]
  Arm Dynamics2/2(Moments) -> [M_arm3]
  Arm Dynamics2/3(Omega_out) -> [Omega3]
  Arm Dynamics2/4(Omega_dot_out) -> [Omega_dot3]
  omega_b2/1 -> Arm Dynamics2/5(omega_b)
  Degrees to Radians3/1 -> Arm Dynamics2/2(Comm Angles (rad))
  Comm Angles (deg)2/1 -> Selector8/1
  Selector8/1 -> Degrees to Radians3/1
  Arm Dynamics2/5(T_FaFb) -> [T3_FaFb]  "T_FaFb3"
  [T3_FaFb] -> Bus Creator/3
  Bus Creator1/1 -> Angles (rad)/1
  [Angles_1] -> Bus Creator1/1
  [Angles_2] -> Bus Creator1/2
  [Angles_3] -> Bus Creator1/3
  Arm Dynamics/6(Angles (rad)) -> [Angles_1]  "Angles Arm 1"
  Arm Dynamics1/6(Angles (rad)) -> [Angles_2]  "Angles Arm 2"
  Arm Dynamics2/6(Angles (rad)) -> [Angles_3]  "Angles Arm 3"
  Arm Dynamics/7(r_p) -> [r_p_1]
  Arm Dynamics1/7(r_p) -> [r_p_2]
  Arm Dynamics2/7(r_p) -> [r_p_3]

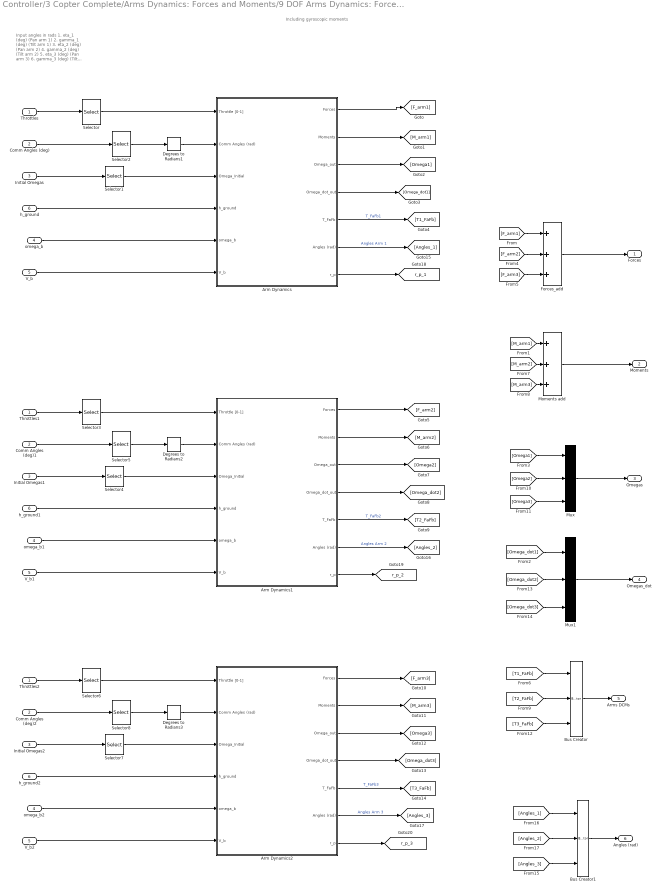
== system Controller/3 Copter Complete/Arms Dynamics: Forces and Moments/9 DOF Arms Dynamics: Forces and Moments/9 DOF Arms Dynamics: Forces and Moments ==
  note: Including gyroscopic moments
  note: Input angles in rads
      |
      | 1. eta_1 (deg)  (Pan arm 1)
      | 2. gamma_1 (deg)  (Tilt arm 1)
      |
      | 3. eta_2 (deg)  (Pan arm 2)
      | 4. gamma_2 (deg)  (Tilt arm 2)
      |
      | 5. eta_3 (deg)  (Pan arm  3)
      | 6. gamma_3 (deg)  (Tilt arm 3)
  Throttles : Inport
  Comm Angles (deg) : Inport  Port=2
  Initial Omegas : Inport  Port=3
  omega_b : Inport  Port=4
  V_b : Inport  Port=5
  h_ground : Inport  Port=6
  Arm Dynamics : Subsystem  AncestorBlock=XXCopter/Arm Dynamics  TreatAsAtomicUnit=on  mask(Arm dynamics, kinematics, forces and moments){Rot_sign=Rotation_sign(1), tau=Tau_motors, arm_hub_pos=l*[1;0;0], arm_axis=[l_arm;0;0], arm_num=1, eta_dir=[1;0;0], gamma_dir=[0;1;0], J_T=J_T, J_FA=J_FA, h=h, Torq_ini=Initial_Torques(1), Omega_ini=Initial_Omegas(1), init_eta=0, init_gamma=0, omega_n=35, xi=1.45, c=0}
      mask prompts: Rot_sign "Rotation sign"; tau "Tau motors"; arm_hub_pos "Arm Hub position"; arm_axis "Arm Hub from servo"; arm_num "Arm number"; eta_dir "eta direcction"; gamma_dir "gamma direction"; J_T "Inertia Motor+prop"; J_FA "Inertia Forearm"; h "h propeller hub"; Torq_ini "Torque Initial Condition"; Omega_ini "Omega Initial Condition"; init_eta "Initial eta  (rad)"; init_gamma "Initial gamma  (rad)"; omega_n "Servo natural frequency"; xi "Servo damping"; c "Derivative param"
      mask help:
      | This block only accepts arms oriented in x-axis or y-axis: eta and gamma directions can only be [1,0,0] or [0,1,0]
      | Note rotations order is [eta (pan) ,gamma (tilt),0]
      |
      | If Arm number 1 (Forward one)
      | eta_dir=[1,0,0]
      | gamma_dir=[0,1,0]
      |
      | If Arm number 2 or 3 (rear ones)
      | eta_dir=[0,1,0]
      | gamma_dir=[1,0,0]
      mask TypeOptions Rot_sign: Aerodynamics Propeller/Rot_sign | Gyroscopic Moments/Rot_sign
      mask TypeOptions tau: ESC+Motor Dynamcis/tau
      mask TypeOptions arm_hub_pos: Arms Kinematics/Arm_hub_position
      mask TypeOptions arm_axis: Gyroscopic Moments/Arm_axis
      mask TypeOptions arm_num: Arms Kinematics/Arm_number
      mask TypeOptions eta_dir: Arms Kinematics/eta_dir | Gyroscopic Moments/eta_dir
      mask TypeOptions gamma_dir: Arms Kinematics/gamma_dir | Gyroscopic Moments/gamma_dir
      mask TypeOptions J_T: ESC+Motor Dynamcis/J_T | Gyroscopic Moments/J_T
      mask TypeOptions J_FA: Gyroscopic Moments/J_FA
      mask TypeOptions h: Arms Kinematics/h_prop
      mask TypeOptions Torq_ini: Initial_torque/X0
      mask TypeOptions Omega_ini: initial_omega/X0
      mask TypeOptions init_eta: Servos Dynamics/init_eta
      mask TypeOptions omega_n: Servos Dynamics/omega_n
      mask TypeOptions xi: Servos Dynamics/xi
      mask TypeOptions c: Servos Dynamics/derv_param
      mask Display:
      | % fprintf(' Arm number %i \n dynamics',arm_num)
      | 
      | 
      | disp(['{\bf \fontsize{16}',sprintf('Arm number\n\n'),num2str(arm_num),sprintf('\n\n Dynamics '),'}'], 'texmode','on');
  Arm Dynamics1 : Subsystem  AncestorBlock=XXCopter/Arm Dynamics  TreatAsAtomicUnit=on  mask(Arm dynamics, kinematics, forces and moments){Rot_sign=Rotation_sign(2), tau=Tau_motors, arm_hub_pos=l*[-1/2;sqrt(3)/2;0], arm_axis=[0;l_arm;0], arm_num=2, eta_dir=[0;1;0], gamma_dir=[1;0;0], J_T=J_T, J_FA=J_FA, h=h, Torq_ini=Initial_Torques(2), Omega_ini=Initial_Omegas(2), init_eta=0, init_gamma=0, omega_n=35, xi=1.45, c=0}
      mask prompts: Rot_sign "Rotation sign"; tau "Tau motors"; arm_hub_pos "Arm Hub position"; arm_axis "Arm Hub from servo"; arm_num "Arm number"; eta_dir "eta direcction"; gamma_dir "gamma direction"; J_T "Inertia Motor+prop"; J_FA "Inertia Forearm"; h "h propeller hub"; Torq_ini "Torque Initial Condition"; Omega_ini "Omega Initial Condition"; init_eta "Initial eta  (rad)"; init_gamma "Initial gamma  (rad)"; omega_n "Servo natural frequency"; xi "Servo damping"; c "Derivative param"
      mask help:
      | This block only accepts arms oriented in x-axis or y-axis: eta and gamma directions can only be [1,0,0] or [0,1,0]
      | Note rotations order is [eta (pan) ,gamma (tilt),0]
      |
      | If Arm number 1 (Forward one)
      | eta_dir=[1,0,0]
      | gamma_dir=[0,1,0]
      |
      | If Arm number 2 or 3 (rear ones)
      | eta_dir=[0,1,0]
      | gamma_dir=[1,0,0]
      mask TypeOptions Rot_sign: Aerodynamics Propeller/Rot_sign | Gyroscopic Moments/Rot_sign
      mask TypeOptions tau: ESC+Motor Dynamcis/tau
      mask TypeOptions arm_hub_pos: Arms Kinematics/Arm_hub_position
      mask TypeOptions arm_axis: Gyroscopic Moments/Arm_axis
      mask TypeOptions arm_num: Arms Kinematics/Arm_number
      mask TypeOptions eta_dir: Arms Kinematics/eta_dir | Gyroscopic Moments/eta_dir
      mask TypeOptions gamma_dir: Arms Kinematics/gamma_dir | Gyroscopic Moments/gamma_dir
      mask TypeOptions J_T: ESC+Motor Dynamcis/J_T | Gyroscopic Moments/J_T
      mask TypeOptions J_FA: Gyroscopic Moments/J_FA
      mask TypeOptions h: Arms Kinematics/h_prop
      mask TypeOptions Torq_ini: Initial_torque/X0
      mask TypeOptions Omega_ini: initial_omega/X0
      mask TypeOptions init_eta: Servos Dynamics/init_eta
      mask TypeOptions omega_n: Servos Dynamics/omega_n
      mask TypeOptions xi: Servos Dynamics/xi
      mask TypeOptions c: Servos Dynamics/derv_param
      mask Display:
      | % fprintf(' Arm number %i \n dynamics',arm_num)
      | 
      | 
      | disp(['{\bf \fontsize{16}',sprintf('Arm number\n\n'),num2str(arm_num),sprintf('\n\n Dynamics '),'}'], 'texmode','on');
  Arm Dynamics2 : Subsystem  AncestorBlock=XXCopter/Arm Dynamics  TreatAsAtomicUnit=on  mask(Arm dynamics, kinematics, forces and moments){Rot_sign=Rotation_sign(3), tau=Tau_motors, arm_hub_pos=l*[-1/2;-sqrt(3)/2;0], arm_axis=[0;-l_arm;0], arm_num=3, eta_dir=[0;1;0], gamma_dir=[1;0;0], J_T=J_T, J_FA=J_FA, h=h, Torq_ini=Initial_Torques(3), Omega_ini=Initial_Omegas(3), init_eta=0, init_gamma=0, omega_n=35, xi=1.45, c=0}
      mask prompts: Rot_sign "Rotation sign"; tau "Tau motors"; arm_hub_pos "Arm Hub position"; arm_axis "Arm Hub from servo"; arm_num "Arm number"; eta_dir "eta direcction"; gamma_dir "gamma direction"; J_T "Inertia Motor+prop"; J_FA "Inertia Forearm"; h "h propeller hub"; Torq_ini "Torque Initial Condition"; Omega_ini "Omega Initial Condition"; init_eta "Initial eta  (rad)"; init_gamma "Initial gamma  (rad)"; omega_n "Servo natural frequency"; xi "Servo damping"; c "Derivative param"
      mask help:
      | This block only accepts arms oriented in x-axis or y-axis: eta and gamma directions can only be [1,0,0] or [0,1,0]
      | Note rotations order is [eta (pan) ,gamma (tilt),0]
      |
      | If Arm number 1 (Forward one)
      | eta_dir=[1,0,0]
      | gamma_dir=[0,1,0]
      |
      | If Arm number 2 or 3 (rear ones)
      | eta_dir=[0,1,0]
      | gamma_dir=[1,0,0]
      mask TypeOptions Rot_sign: Aerodynamics Propeller/Rot_sign | Gyroscopic Moments/Rot_sign
      mask TypeOptions tau: ESC+Motor Dynamcis/tau
      mask TypeOptions arm_hub_pos: Arms Kinematics/Arm_hub_position
      mask TypeOptions arm_axis: Gyroscopic Moments/Arm_axis
      mask TypeOptions arm_num: Arms Kinematics/Arm_number
      mask TypeOptions eta_dir: Arms Kinematics/eta_dir | Gyroscopic Moments/eta_dir
      mask TypeOptions gamma_dir: Arms Kinematics/gamma_dir | Gyroscopic Moments/gamma_dir
      mask TypeOptions J_T: ESC+Motor Dynamcis/J_T | Gyroscopic Moments/J_T
      mask TypeOptions J_FA: Gyroscopic Moments/J_FA
      mask TypeOptions h: Arms Kinematics/h_prop
      mask TypeOptions Torq_ini: Initial_torque/X0
      mask TypeOptions Omega_ini: initial_omega/X0
      mask TypeOptions init_eta: Servos Dynamics/init_eta
      mask TypeOptions omega_n: Servos Dynamics/omega_n
      mask TypeOptions xi: Servos Dynamics/xi
      mask TypeOptions c: Servos Dynamics/derv_param
      mask Display:
      | % fprintf(' Arm number %i \n dynamics',arm_num)
      | 
      | 
      | disp(['{\bf \fontsize{16}',sprintf('Arm number\n\n'),num2str(arm_num),sprintf('\n\n Dynamics '),'}'], 'texmode','on');
  Bus Creator : BusCreator  Inputs=3
  Bus Creator1 : BusCreator  Inputs=3
  Comm Angles (deg)1 : InportShadow  Port=2
  Comm Angles (deg)2 : InportShadow  Port=2
  Degrees to Radians1 : simulink_extras/Transformations/Degrees to Radians
  Degrees to Radians2 : simulink_extras/Transformations/Degrees to Radians
  Degrees to Radians3 : simulink_extras/Transformations/Degrees to Radians
  Forces_add : Sum  Inputs=+++
  Initial Omegas1 : InportShadow  Port=3
  Initial Omegas2 : InportShadow  Port=3
  Moments add : Sum  Inputs=+++
  Mux : Mux  Inputs=3
  Mux1 : Mux  Inputs=3
  Selector : Selector  InputPortWidth=3  Indices=[1]
  Selector1 : Selector  InputPortWidth=3  Indices=[1]
  Selector2 : Selector  InputPortWidth=6  Indices=[1,2]
  Selector3 : Selector  InputPortWidth=3  Indices=2
  Selector4 : Selector  InputPortWidth=3  Indices=2
  Selector5 : Selector  InputPortWidth=6  Indices=[3,4]
  Selector6 : Selector  InputPortWidth=3  Indices=3
  Selector7 : Selector  InputPortWidth=3  Indices=3
  Selector8 : Selector  InputPortWidth=6  Indices=[5,6]
  Throttles1 : InportShadow
  Throttles2 : InportShadow
  V_b1 : InportShadow  Port=5
  V_b2 : InportShadow  Port=5
  h_ground1 : InportShadow  Port=6
  h_ground2 : InportShadow  Port=6
  omega_b1 : InportShadow  Port=4
  omega_b2 : InportShadow  Port=4
  Forces : Outport
  Moments : Outport  Port=2
  Omegas : Outport  Port=3
  Omegas_dot : Outport  Port=4
  Arms DCMs : Outport  Port=5
  Angles (rad) : Outport  Port=6
  tag scope: r_p_1=global, r_p_2=global, r_p_3=global
  wires:
  Selector1/1 -> Arm Dynamics/3(Omega_Initial)
  Throttles/1 -> Selector/1
  Initial Omegas/1 -> Selector1/1
  Selector/1 -> Arm Dynamics/1(Throttle [0-1])
  V_b/1 -> Arm Dynamics/6(V_b)
  Forces_add/1 -> Forces/1
  Moments add/1 -> Moments/1
  Mux/1 -> Omegas/1
  Mux1/1 -> Omegas_dot/1
  h_ground/1 -> Arm Dynamics/4(h_ground)
  Arm Dynamics/1(Forces) -> [F_arm1]
  Arm Dynamics/2(Moments) -> [M_arm1]
  Arm Dynamics/3(Omega_out) -> [Omega1]
  Arm Dynamics/4(Omega_dot_out) -> [Omega_dot1]
  [F_arm1] -> Forces_add/1
  [M_arm1] -> Moments add/1
  [Omega_dot1] -> Mux1/1
  [Omega1] -> Mux/1
  omega_b/1 -> Arm Dynamics/5(omega_b)
  [F_arm2] -> Forces_add/2
  [F_arm3] -> Forces_add/3
  [Omega2] -> Mux/2
  [Omega3] -> Mux/3
  [Omega_dot2] -> Mux1/2
  [Omega_dot3] -> Mux1/3
  [M_arm3] -> Moments add/3
  [M_arm2] -> Moments add/2
  Degrees to Radians1/1 -> Arm Dynamics/2(Comm Angles (rad))
  Comm Angles (deg)/1 -> Selector2/1
  Selector2/1 -> Degrees to Radians1/1
  Arm Dynamics/5(T_FaFb) -> [T1_FaFb]  "T_FaFb1"
  Bus Creator/1 -> Arms DCMs/1
  [T1_FaFb] -> Bus Creator/1
  Selector4/1 -> Arm Dynamics1/3(Omega_Initial)
  Throttles1/1 -> Selector3/1
  Initial Omegas1/1 -> Selector4/1
  Selector3/1 -> Arm Dynamics1/1(Throttle [0-1])
  V_b1/1 -> Arm Dynamics1/6(V_b)
  h_ground1/1 -> Arm Dynamics1/4(h_ground)
  Arm Dynamics1/1(Forces) -> [F_arm2]
  Arm Dynamics1/2(Moments) -> [M_arm2]
  Arm Dynamics1/3(Omega_out) -> [Omega2]
  Arm Dynamics1/4(Omega_dot_out) -> [Omega_dot2]
  omega_b1/1 -> Arm Dynamics1/5(omega_b)
  Degrees to Radians2/1 -> Arm Dynamics1/2(Comm Angles (rad))
  Comm Angles (deg)1/1 -> Selector5/1
  Selector5/1 -> Degrees to Radians2/1
  Arm Dynamics1/5(T_FaFb) -> [T2_FaFb]  "T_FaFb2"
  [T2_FaFb] -> Bus Creator/2
  Selector7/1 -> Arm Dynamics2/3(Omega_Initial)
  Throttles2/1 -> Selector6/1
  Initial Omegas2/1 -> Selector7/1
  Selector6/1 -> Arm Dynamics2/1(Throttle [0-1])
  V_b2/1 -> Arm Dynamics2/6(V_b)
  h_ground2/1 -> Arm Dynamics2/4(h_ground)
  Arm Dynamics2/1(Forces) -> [F_arm3]
  Arm Dynamics2/2(Moments) -> [M_arm3]
  Arm Dynamics2/3(Omega_out) -> [Omega3]
  Arm Dynamics2/4(Omega_dot_out) -> [Omega_dot3]
  omega_b2/1 -> Arm Dynamics2/5(omega_b)
  Degrees to Radians3/1 -> Arm Dynamics2/2(Comm Angles (rad))
  Comm Angles (deg)2/1 -> Selector8/1
  Selector8/1 -> Degrees to Radians3/1
  Arm Dynamics2/5(T_FaFb) -> [T3_FaFb]  "T_FaFb3"
  [T3_FaFb] -> Bus Creator/3
  Bus Creator1/1 -> Angles (rad)/1
  [Angles_1] -> Bus Creator1/1
  [Angles_2] -> Bus Creator1/2
  [Angles_3] -> Bus Creator1/3
  Arm Dynamics/6(Angles (rad)) -> [Angles_1]  "Angles Arm 1"
  Arm Dynamics1/6(Angles (rad)) -> [Angles_2]  "Angles Arm 2"
  Arm Dynamics2/6(Angles (rad)) -> [Angles_3]  "Angles Arm 3"
  Arm Dynamics/7(r_p) -> [r_p_1]
  Arm Dynamics1/7(r_p) -> [r_p_2]
  Arm Dynamics2/7(r_p) -> [r_p_3]
